simulink model "lab3_prob2_rd3"  (R2024a)
settings: Solver=VariableStepAuto  StartTime=0.0  StopTime=20  RelTol=1e-3
values from neighbouring files (symbols this model uses):
  G2G3G4H3_den = conv(TF_G3G4H3_den, G_den2)    [Problem2_Aldovino_Bejasa.m]
  G2G3G4H3_num = conv(TF_G3G4H3_num, G_num2)    [Problem2_Aldovino_Bejasa.m]
  G_den1 = [1 0 0]    [Problem2_Aldovino_Bejasa.m]
  G_den4 = [0 2 0]    [Problem2_Aldovino_Bejasa.m]
  G_num1 = [1]    [Problem2_Aldovino_Bejasa.m]
  G_num4 = [1]    [Problem2_Aldovino_Bejasa.m]
  H_den1 = [1 0]    [Problem2_Aldovino_Bejasa.m]
  H_den2 = [1 -1]    [Problem2_Aldovino_Bejasa.m]
  H_num1 = [1]    [Problem2_Aldovino_Bejasa.m]
  H_num2 = [1]    [Problem2_Aldovino_Bejasa.m]
settings Model: Creator=HUAWEI  LastModifiedBy=HUAWEI

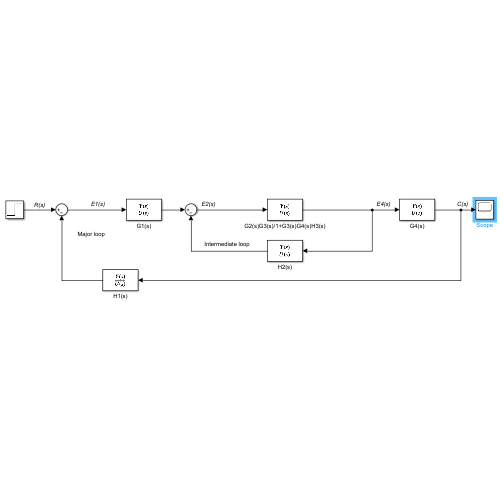
[thumbnail: Simulink's stored preview of the top-level diagram]
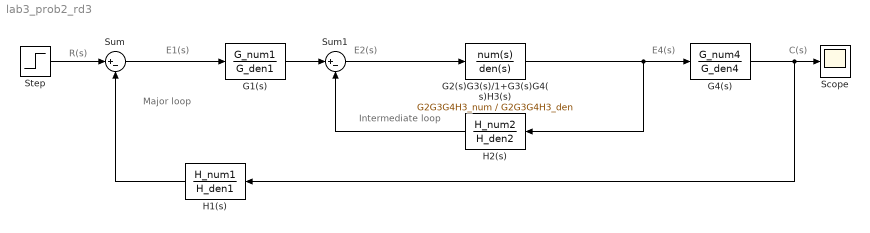
== system lab3_prob2_rd3 ==
  note: Major loop
  note: C(s)
  note: E4(s)
  note: E1(s)
  note: Intermediate loop
  note: R(s)
  note: E2(s)
  G1(s) : TransferFcn  Numerator=G_num1  Denominator=G_den1
  G2(s)G3(s)/1+G3(s)G4(s)H3(s) : TransferFcn  Numerator=G2G3G4H3_num  Denominator=G2G3G4H3_den
  G4(s) : TransferFcn  Numerator=G_num4  Denominator=G_den4
  H1(s) : TransferFcn  Numerator=H_num1  Denominator=H_den1
  H2(s) : TransferFcn  Numerator=H_num2  Denominator=H_den2
  Scope : Scope
  Step : Step  Time=0  SampleTime=0
  Sum : Sum  Inputs=|+-
  Sum1 : Sum  Inputs=|+-
  wires:
  H1(s)/1 -> Sum/2
  G2(s)G3(s)/1+G3(s)G4(s)H3(s)/1 -> H2(s)/1, G4(s)/1
  Sum1/1 -> G2(s)G3(s)/1+G3(s)G4(s)H3(s)/1
  G1(s)/1 -> Sum1/1
  H2(s)/1 -> Sum1/2
  G4(s)/1 -> H1(s)/1, Scope/1
  Step/1 -> Sum/1
  Sum/1 -> G1(s)/1
